simulink model "lab8task4Remastered"  (Simulink 7.5)
settings: Solver=ode45  StartTime=0.0  StopTime=100  RelTol=1e-3
undefined symbols (not defined in the file or in its folder): DiscIntNeverNeededParam
settings Model: Creator=Dranik_win  LastModifiedBy=Dranik_win

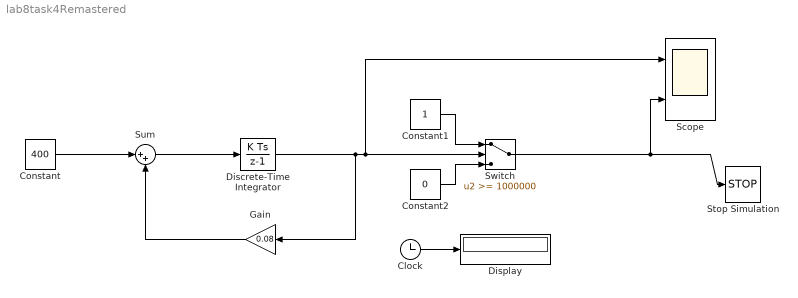
== system lab8task4Remastered ==
  Clock : Clock
      settings: Decimation=10
  Constant : Constant  Value=400  OutDataType=fixdt(1, 16)  OutScaling=2^0
  Constant1 : Constant  OutDataType=fixdt(1, 16)  OutScaling=2^0
  Constant2 : Constant  Value=0  OutDataType=fixdt(1, 16)  OutScaling=2^0
  Discrete-Time Integrator : DiscreteIntegrator  OutDataType=fixdt(1, 16)  OutScaling=2^0  ICPrevOutput=DiscIntNeverNeededParam  ICPrevScaledInput=DiscIntNeverNeededParam
  Display : Display
  Gain : Gain  Gain=0.08  ParameterDataType=fixdt(1, 16)  ParameterScaling=2^0  OutDataType=fixdt(1, 16)  OutScaling=2^0
  Scope : Scope  NumInputPorts=2
      settings: YMin=-5~-5  YMax=5~5
  Stop Simulation : Stop
  Sum : Sum  Inputs=|++  OutDataType=fixdt(1, 16)  OutScaling=2^0
  Switch : Switch  Threshold=1000000  OutDataType=fixdt(1, 16)  OutScaling=2^0
  wires:
  Sum/1 -> Discrete-Time Integrator/1
  Constant/1 -> Sum/1
  Discrete-Time Integrator/1 -> Gain/1, Switch/2, Scope/1
  Gain/1 -> Sum/2
  Clock/1 -> Display/1
  Constant1/1 -> Switch/1
  Constant2/1 -> Switch/3
  Switch/1 -> Scope/2, Stop Simulation/1
